simulink model "RadarSimulinkProjectRev011"  (R2024a)
settings: Solver=VariableStepAuto  StartTime=0.0  StopTime=0.0125*2  RelTol=1e-3
values from neighbouring files (symbols this model uses):
  AngleTime = SweepTime/10    (= 10000)    [InitializationOfVariablesRev000.m]    (also in InitializationOfVariablesRev001.m; InitializationOfVariablesRev002.m = 2000; InitializationOfVariablesRev003.m = 20000; InitializationOfVariablesRev004.m = 2097152)
  ASR_LUT = Rsamp    [InitializationOfVariablesRev003.m]    (also in InitializationOfVariablesRev004.m = round((R*2*SystemFs)/c); InitializationOfVariablesRev005.m = round((R*2*SystemFs)/c))
  Btn_Debounce = 20000    [InitializationOfVariablesRev003.m]    (also in InitializationOfVariablesRev004.m; InitializationOfVariablesRev005.m)
  ChirpNc = 128    [InitializationOfVariablesRev004.m]    (also in InitializationOfVariablesRev005.m)
  ChirpSizeLength = length(FCW)    [InitializationOfVariablesRev004.m]    (also in InitializationOfVariablesRev005.m = 16384)
  DeciFactor = 8    [InitializationOfVariablesRev005.m]
  FCW = [FCW_p1, FCW_p2]    [InitializationOfVariablesRev002.m]    (also in InitializationOfVariablesRev003.m; InitializationOfVariablesRev004.m = interp1(1:length(FCW_base), FCW_base,      linspace(1, lengt; InitializationOfVariablesRev005.m = f / SystemFs)
  RXFFTLength = 4096    [InitializationOfVariablesRev003.m]    (also in InitializationOfVariablesRev004.m = 1024; InitializationOfVariablesRev005.m = 2048)
  SweepTime = 100000    [InitializationOfVariablesRev000.m]    (also in InitializationOfVariablesRev001.m; InitializationOfVariablesRev002.m = 20000; InitializationOfVariablesRev003.m = 200000; InitializationOfVariablesRev004.m = 23068672)
undefined symbols (not defined in the file or in its folder): SignalGenerationForAnalysis, Subsystem, xc7a200tfbg676
libraries: hdlBasic x453, hdlUtilities x11, hdlDSPIP x11, vmcUtilities x1
(part 4 of 5)

== system RadarSimulinkProjectRev011/RangeProcessing/DC Removal3 ==
  note: Measured delay between DC removal and RAM delay, offset by 54 (apparently)
  DataIN : Inport
  tlast : Inport  Port=2
  tready : Inport  Port=3
  Accumulator : hdlBasic/Accumulator  operation=Add  n_bits=64  overflow=Wrap  scale=1  rst=on  hasbypass=off  en=on  latency=1  msb_inp=100  msb=100  lsb=-100  use_behavioral_HDL=on  implementation=Fabric  XmcBlockStatus=1  maskContainerNames=group3  block_type=accum  block_config=sysgen:Accum_config  block_width=566  block_height=845
  AddSub : hdlBasic/AddSub  mode=Subtraction  use_carryin=off  use_carryout=off  en=off  latency=1  precision=Full  arith_type=Unsigned  n_bits=16  bin_pt=14  quantization=Truncate  overflow=Wrap  use_behavioral_HDL=off  hw_selection=Fabric  pipelined=off  XmcBlockStatus=1  maskContainerNames=tabcontainer1  block_type=addsub  block_config=sysgen:Addsub_config
  Constant : hdlBasic/Constant  const=ChirpSizeLength-1  gui_display_data_type=Fixed-point  arith_type=Signed (2's comp)  n_bits=16  bin_pt=0  preci_type=Single  exp_width=8  frac_width=24  explicit_period=on  period=P1  XmcBlockStatus=1  maskContainerNames=tabcontainer1  block_type=constant  block_config=sysgen:Constant_config
  Constant1 : hdlBasic/Constant  const=ChirpSizeLength-1  gui_display_data_type=Fixed-point  arith_type=Signed (2's comp)  n_bits=16  bin_pt=0  preci_type=Single  exp_width=8  frac_width=24  explicit_period=off  period=1  XmcBlockStatus=1  maskContainerNames=tabcontainer1  block_type=constant  block_config=sysgen:Constant_config
  Convert10 : hdlBasic/Convert  gui_display_data_type=Fixed-point  arith_type=Signed (2's comp)  n_bits=32  bin_pt=16  float_type=Single  exp_bits=8  fraction_bits=24  quantization="Round  (unbiased: Even Values)"  overflow=Saturate  en=off  latency=1  pipeline=off  XmcBlockStatus=1  maskContainerNames=group2  block_type=convert  block_config=sysgen:Convert_config  block_width=595  block_height=885
  Counter : hdlBasic/Counter  cnt_type=Count limited  cnt_to=ChirpSizeLength-1  operation=Up  start_count=0  cnt_by_val=1  arith_type=Unsigned  n_bits=14  bin_pt=0  load_pin=off  rst=on  en=on  explicit_period=Explicit  period=P1  use_behavioral_HDL=off  implementation=Fabric  XmcBlockStatus=1  maskContainerNames=group1  block_type=counter  block_config=sysgen:Counter_config  block_width=531  block_height=1023
  Counter1 : hdlBasic/Counter  cnt_type=Count limited  cnt_to=ChirpSizeLength-1  operation=Up  start_count=0  cnt_by_val=1  arith_type=Unsigned  n_bits=14  bin_pt=0  load_pin=off  rst=on  en=on  explicit_period=Explicit  period=P1  use_behavioral_HDL=off  implementation=Fabric  XmcBlockStatus=1  maskContainerNames=group1  block_type=counter  block_config=sysgen:Counter_config  block_width=531  block_height=1023
  Delay1 : hdlBasic/Delay  rst=off  en=off  latency=72  reg_retiming=off  XmcBlockStatus=1  maskContainerNames=group1  block_type=delay  block_config=sysgen:Delay_config
  Delay2 : hdlBasic/Delay  rst=off  en=off  latency=55  reg_retiming=off  XmcBlockStatus=1  maskContainerNames=group1  block_type=delay  block_config=sysgen:Delay_config
  Divide : hdlBasic/Divide  flow_control=NonBlocking  axi_optimize_goal=Resources  algorithm_type=Radix2  fractional_width=32  latency=1  rate=1  has_a_tlast=off  has_a_tuser=off  has_b_tlast=off  has_b_tuser=off  en=off  has_result_tready=off  result_tlast_behv=Pass_A_TLAST  has_underflow=off  has_overflow=off  has_invalid_op=off  has_divide_by_zero=off  fpo_op_type=mergeddivide  XmcBlockStatus=1  maskContainerNames=tabcontainer1  block_type=divide  block_config=sysgen:FPOBlockDescriptor_config
  Register : hdlBasic/Register  init=0  rst=off  en=on  XmcBlockStatus=1  maskContainerNames=tabcontainer1  block_type=register  block_config=sysgen:Register_config
  Relational : hdlBasic/Relational  mode=a=b  op_type=Bool  en=off  latency=0  XmcBlockStatus=1  maskContainerNames=tabcontainer1  block_type=relational  block_config=sysgen:Relational_config
  Simple Dual Port RAM : hdlBasic/Simple Dual Port RAM  depth=ChirpSizeLength  initVector=0  distributed_mem=Distributed memory  init_b=0  rst_b=off  en_a=off  en_b=off  latency=1  write_mode_B=Read After Write  explicit_period=[]  period=[]  simulation_type=fast_sim  XmcBlockStatus=1  maskContainerNames=tabcontainer1  block_type=sdpram  block_config=sysgen:Sdpram_config  optimize=Area
      settings: infoedit=[]
  Simple Dual Port RAM1 : hdlBasic/Simple Dual Port RAM  depth=ChirpSizeLength  initVector=0  distributed_mem=Distributed memory  init_b=0  rst_b=off  en_a=off  en_b=off  latency=1  write_mode_B=Read After Write  explicit_period=[]  period=[]  simulation_type=fast_sim  XmcBlockStatus=1  maskContainerNames=tabcontainer1  block_type=sdpram  block_config=sysgen:Sdpram_config  optimize=Area
      settings: infoedit=[]
  DataOUT : Outport
  treadyOUT : Outport  Port=2
  wires:
  Accumulator/1 -> Register/1
  Register/1 -> Divide/1
  AddSub/1 -> Convert10/1
  Constant/1 -> Divide/2
  Counter/1 -> Simple Dual Port RAM1/1, Simple Dual Port RAM/1, Relational/2
  Counter1/1 -> Simple Dual Port RAM1/4, Simple Dual Port RAM/4
  Constant1/1 -> Relational/1
  Simple Dual Port RAM/1 -> Delay1/1
  Simple Dual Port RAM1/1 -> Delay2/1
  Delay2/1 -> treadyOUT/1
  Convert10/1 -> DataOUT/1
  Delay1/1 -> AddSub/1
  Divide/1 -> AddSub/2
  DataIN/1 -> Accumulator/1, Simple Dual Port RAM/2
  tready/1 -> Accumulator/3, Counter1/2, Simple Dual Port RAM1/3, Simple Dual Port RAM1/2, Simple Dual Port RAM/3, Counter/2
  tlast/1 -> Register/2, Accumulator/2, Counter/1
  Relational/1 -> Counter1/1

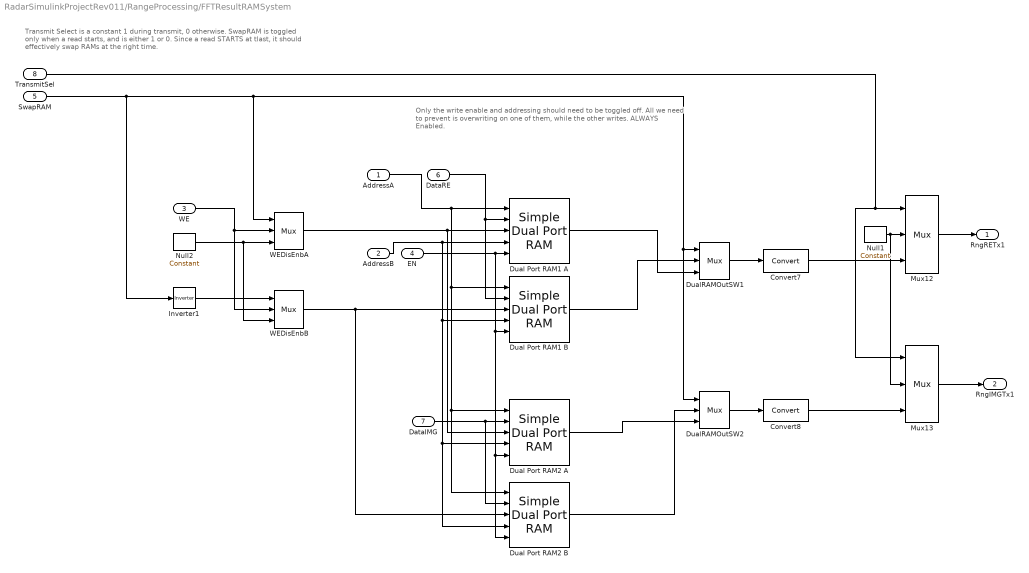
== system RadarSimulinkProjectRev011/RangeProcessing/FFTResultRAMSystem ==
  note: Transmit Select is a constant 1 during transmit, 0 otherwise.
      | SwapRAM is toggled only when a read starts, and is either 1 or 0.
      | Since a read STARTS at tlast, it should effectively swap RAMs at the right time.
  note: Only the write enable and addressing should need to be toggled off.
      | All we need to prevent is overwriting on one of them, while the other writes.
      | ALWAYS Enabled.
  AddressA : Inport
  AddressB : Inport  Port=2
  WE : Inport  Port=3
  EN : Inport  Port=4
  SwapRAM : Inport  Port=5
  DataRE : Inport  Port=6
  DataIMG : Inport  Port=7
  TransmitSel : Inport  Port=8
  Convert7 : hdlBasic/Convert  gui_display_data_type=Fixed-point  arith_type="Signed  (2's comp)"  n_bits=17  bin_pt=16  float_type=Single  exp_bits=8  fraction_bits=24  quantization=Truncate  overflow=Saturate  en=off  latency=0  pipeline=off  XmcBlockStatus=1  maskContainerNames=group2  block_type=convert  block_config=sysgen:Convert_config  block_width=595  block_height=885
  Convert8 : hdlBasic/Convert  gui_display_data_type=Fixed-point  arith_type="Signed  (2's comp)"  n_bits=17  bin_pt=16  float_type=Single  exp_bits=8  fraction_bits=24  quantization=Truncate  overflow=Saturate  en=off  latency=0  pipeline=off  XmcBlockStatus=1  maskContainerNames=group2  block_type=convert  block_config=sysgen:Convert_config  block_width=595  block_height=885
  Dual Port RAM1 A : hdlBasic/Simple Dual Port RAM  depth=ChirpNc*RXFFTLength  initVector=0  distributed_mem=Distributed memory  init_b=0  rst_b=off  en_a=on  en_b=off  latency=1  write_mode_B=Read After Write  explicit_period=[]  period=[]  simulation_type=fast_sim  XmcBlockStatus=1  maskContainerNames=tabcontainer1  block_type=sdpram  block_config=sysgen:Sdpram_config  optimize=Area
      settings: infoedit=[]
  Dual Port RAM1 B : hdlBasic/Simple Dual Port RAM  depth=ChirpNc*RXFFTLength  initVector=0  distributed_mem=Distributed memory  init_b=0  rst_b=off  en_a=on  en_b=off  latency=1  write_mode_B=Read After Write  explicit_period=[]  period=[]  simulation_type=fast_sim  XmcBlockStatus=1  maskContainerNames=tabcontainer1  block_type=sdpram  block_config=sysgen:Sdpram_config  optimize=Area
      settings: infoedit=[]
  Dual Port RAM2 A : hdlBasic/Simple Dual Port RAM  depth=ChirpNc*RXFFTLength  initVector=0  distributed_mem=Distributed memory  init_b=0  rst_b=off  en_a=on  en_b=off  latency=1  write_mode_B=Read After Write  explicit_period=[]  period=[]  simulation_type=fast_sim  XmcBlockStatus=1  maskContainerNames=tabcontainer1  block_type=sdpram  block_config=sysgen:Sdpram_config  optimize=Area
      settings: infoedit=[]
  Dual Port RAM2 B : hdlBasic/Simple Dual Port RAM  depth=ChirpNc*RXFFTLength  initVector=0  distributed_mem=Distributed memory  init_b=0  rst_b=off  en_a=on  en_b=off  latency=1  write_mode_B=Read After Write  explicit_period=[]  period=[]  simulation_type=fast_sim  XmcBlockStatus=1  maskContainerNames=tabcontainer1  block_type=sdpram  block_config=sysgen:Sdpram_config  optimize=Area
      settings: infoedit=[]
  DualRAMOutSW1 : hdlBasic/Mux  inputs=2  en=off  latency=0  precision=Full  arith_type=Unsigned  n_bits=16  bin_pt=14  quantization=Truncate  overflow=Wrap  XmcBlockStatus=1  maskContainerNames=tabcontainer1  block_type=mux  block_config=sysgen:Mux_config
  DualRAMOutSW2 : hdlBasic/Mux  inputs=2  en=off  latency=0  precision=Full  arith_type=Unsigned  n_bits=16  bin_pt=14  quantization=Truncate  overflow=Wrap  XmcBlockStatus=1  maskContainerNames=tabcontainer1  block_type=mux  block_config=sysgen:Mux_config
  Inverter1 : hdlBasic/Inverter  en=off  latency=0  XmcBlockStatus=1  maskContainerNames=group2  block_type=inv  block_config=sysgen:Inverter_config
  Mux12 : hdlBasic/Mux  inputs=2  en=off  latency=0  precision=Full  arith_type=Unsigned  n_bits=16  bin_pt=14  quantization=Truncate  overflow=Wrap  XmcBlockStatus=1  maskContainerNames=tabcontainer1  block_type=mux  block_config=sysgen:Mux_config
  Mux13 : hdlBasic/Mux  inputs=2  en=off  latency=0  precision=Full  arith_type=Unsigned  n_bits=16  bin_pt=14  quantization=Truncate  overflow=Wrap  XmcBlockStatus=1  maskContainerNames=tabcontainer1  block_type=mux  block_config=sysgen:Mux_config
  Null1 : hdlBasic/Constant  const=0  gui_display_data_type=Fixed-point  arith_type=Signed (2's comp)  n_bits=16  bin_pt=15  preci_type=Single  exp_width=8  frac_width=24  explicit_period=on  period=P2  XmcBlockStatus=1  maskContainerNames=tabcontainer1  block_type=constant  block_config=sysgen:Constant_config
  Null2 : hdlBasic/Constant  const=0  gui_display_data_type=Boolean  arith_type=Boolean  n_bits=16  bin_pt=15  preci_type=Single  exp_width=8  frac_width=24  explicit_period=on  period=P2  XmcBlockStatus=1  maskContainerNames=tabcontainer1  block_type=constant  block_config=sysgen:Constant_config
  WEDisEnbA : hdlBasic/Mux  inputs=2  en=off  latency=0  precision=Full  arith_type=Unsigned  n_bits=16  bin_pt=14  quantization=Truncate  overflow=Wrap  XmcBlockStatus=1  maskContainerNames=tabcontainer1  block_type=mux  block_config=sysgen:Mux_config
  WEDisEnbB : hdlBasic/Mux  inputs=2  en=off  latency=0  precision=Full  arith_type=Unsigned  n_bits=16  bin_pt=14  quantization=Truncate  overflow=Wrap  XmcBlockStatus=1  maskContainerNames=tabcontainer1  block_type=mux  block_config=sysgen:Mux_config
  RngRETx1 : Outport
  RngIMGTx1 : Outport  Port=2
  wires:
  Mux13/1 -> RngIMGTx1/1
  Mux12/1 -> RngRETx1/1
  Convert8/1 -> Mux13/3
  Convert7/1 -> Mux12/3
  TransmitSel/1 -> Mux12/1, Mux13/1
  Dual Port RAM2 A/1 -> DualRAMOutSW2/3
  Dual Port RAM1 A/1 -> DualRAMOutSW1/3
  Null1/1 -> Mux13/2, Mux12/2
  Dual Port RAM1 B/1 -> DualRAMOutSW1/2
  DualRAMOutSW1/1 -> Convert7/1
  DataRE/1 -> Dual Port RAM1 B/2, Dual Port RAM1 A/2
  DataIMG/1 -> Dual Port RAM2 B/2, Dual Port RAM2 A/2
  EN/1 -> Dual Port RAM1 A/5, Dual Port RAM1 B/5, Dual Port RAM2 B/5, Dual Port RAM2 A/5
  Null2/1 -> WEDisEnbB/3, WEDisEnbA/3
  Dual Port RAM2 B/1 -> DualRAMOutSW2/2
  DualRAMOutSW2/1 -> Convert8/1
  WE/1 -> WEDisEnbB/2, WEDisEnbA/2
  AddressA/1 -> Dual Port RAM1 A/1, Dual Port RAM1 B/1, Dual Port RAM2 A/1, Dual Port RAM2 B/1
  AddressB/1 -> Dual Port RAM2 A/4, Dual Port RAM2 B/4, Dual Port RAM1 B/4, Dual Port RAM1 A/4
  Inverter1/1 -> WEDisEnbB/1
  SwapRAM/1 -> Inverter1/1, WEDisEnbA/1, DualRAMOutSW2/1, DualRAMOutSW1/1
  WEDisEnbA/1 -> Dual Port RAM2 A/3, Dual Port RAM1 A/3
  WEDisEnbB/1 -> Dual Port RAM2 B/3, Dual Port RAM1 B/3

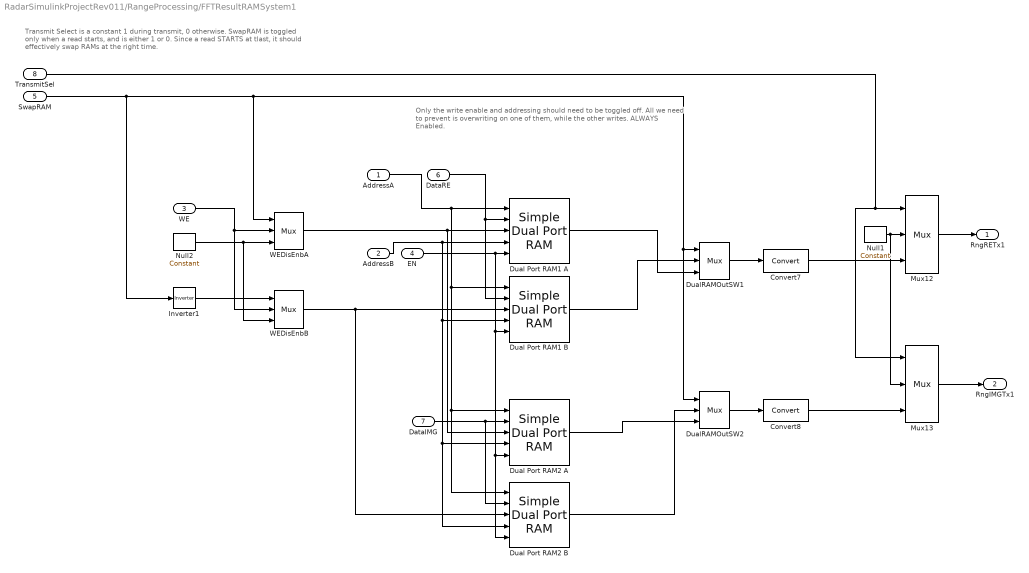
== system RadarSimulinkProjectRev011/RangeProcessing/FFTResultRAMSystem1 ==
  note: Transmit Select is a constant 1 during transmit, 0 otherwise.
      | SwapRAM is toggled only when a read starts, and is either 1 or 0.
      | Since a read STARTS at tlast, it should effectively swap RAMs at the right time.
  note: Only the write enable and addressing should need to be toggled off.
      | All we need to prevent is overwriting on one of them, while the other writes.
      | ALWAYS Enabled.
  AddressA : Inport
  AddressB : Inport  Port=2
  WE : Inport  Port=3
  EN : Inport  Port=4
  SwapRAM : Inport  Port=5
  DataRE : Inport  Port=6
  DataIMG : Inport  Port=7
  TransmitSel : Inport  Port=8
  Convert7 : hdlBasic/Convert  gui_display_data_type=Fixed-point  arith_type="Signed  (2's comp)"  n_bits=17  bin_pt=16  float_type=Single  exp_bits=8  fraction_bits=24  quantization=Truncate  overflow=Saturate  en=off  latency=0  pipeline=off  XmcBlockStatus=1  maskContainerNames=group2  block_type=convert  block_config=sysgen:Convert_config  block_width=595  block_height=885
  Convert8 : hdlBasic/Convert  gui_display_data_type=Fixed-point  arith_type="Signed  (2's comp)"  n_bits=17  bin_pt=16  float_type=Single  exp_bits=8  fraction_bits=24  quantization=Truncate  overflow=Saturate  en=off  latency=0  pipeline=off  XmcBlockStatus=1  maskContainerNames=group2  block_type=convert  block_config=sysgen:Convert_config  block_width=595  block_height=885
  Dual Port RAM1 A : hdlBasic/Simple Dual Port RAM  depth=ChirpNc*RXFFTLength  initVector=0  distributed_mem=Distributed memory  init_b=0  rst_b=off  en_a=on  en_b=off  latency=1  write_mode_B=Read After Write  explicit_period=[]  period=[]  simulation_type=fast_sim  XmcBlockStatus=1  maskContainerNames=tabcontainer1  block_type=sdpram  block_config=sysgen:Sdpram_config  optimize=Area
      settings: infoedit=[]
  Dual Port RAM1 B : hdlBasic/Simple Dual Port RAM  depth=ChirpNc*RXFFTLength  initVector=0  distributed_mem=Distributed memory  init_b=0  rst_b=off  en_a=on  en_b=off  latency=1  write_mode_B=Read After Write  explicit_period=[]  period=[]  simulation_type=fast_sim  XmcBlockStatus=1  maskContainerNames=tabcontainer1  block_type=sdpram  block_config=sysgen:Sdpram_config  optimize=Area
      settings: infoedit=[]
  Dual Port RAM2 A : hdlBasic/Simple Dual Port RAM  depth=ChirpNc*RXFFTLength  initVector=0  distributed_mem=Distributed memory  init_b=0  rst_b=off  en_a=on  en_b=off  latency=1  write_mode_B=Read After Write  explicit_period=[]  period=[]  simulation_type=fast_sim  XmcBlockStatus=1  maskContainerNames=tabcontainer1  block_type=sdpram  block_config=sysgen:Sdpram_config  optimize=Area
      settings: infoedit=[]
  Dual Port RAM2 B : hdlBasic/Simple Dual Port RAM  depth=ChirpNc*RXFFTLength  initVector=0  distributed_mem=Distributed memory  init_b=0  rst_b=off  en_a=on  en_b=off  latency=1  write_mode_B=Read After Write  explicit_period=[]  period=[]  simulation_type=fast_sim  XmcBlockStatus=1  maskContainerNames=tabcontainer1  block_type=sdpram  block_config=sysgen:Sdpram_config  optimize=Area
      settings: infoedit=[]
  DualRAMOutSW1 : hdlBasic/Mux  inputs=2  en=off  latency=0  precision=Full  arith_type=Unsigned  n_bits=16  bin_pt=14  quantization=Truncate  overflow=Wrap  XmcBlockStatus=1  maskContainerNames=tabcontainer1  block_type=mux  block_config=sysgen:Mux_config
  DualRAMOutSW2 : hdlBasic/Mux  inputs=2  en=off  latency=0  precision=Full  arith_type=Unsigned  n_bits=16  bin_pt=14  quantization=Truncate  overflow=Wrap  XmcBlockStatus=1  maskContainerNames=tabcontainer1  block_type=mux  block_config=sysgen:Mux_config
  Inverter1 : hdlBasic/Inverter  en=off  latency=0  XmcBlockStatus=1  maskContainerNames=group2  block_type=inv  block_config=sysgen:Inverter_config
  Mux12 : hdlBasic/Mux  inputs=2  en=off  latency=0  precision=Full  arith_type=Unsigned  n_bits=16  bin_pt=14  quantization=Truncate  overflow=Wrap  XmcBlockStatus=1  maskContainerNames=tabcontainer1  block_type=mux  block_config=sysgen:Mux_config
  Mux13 : hdlBasic/Mux  inputs=2  en=off  latency=0  precision=Full  arith_type=Unsigned  n_bits=16  bin_pt=14  quantization=Truncate  overflow=Wrap  XmcBlockStatus=1  maskContainerNames=tabcontainer1  block_type=mux  block_config=sysgen:Mux_config
  Null1 : hdlBasic/Constant  const=0  gui_display_data_type=Fixed-point  arith_type=Signed (2's comp)  n_bits=16  bin_pt=15  preci_type=Single  exp_width=8  frac_width=24  explicit_period=on  period=P2  XmcBlockStatus=1  maskContainerNames=tabcontainer1  block_type=constant  block_config=sysgen:Constant_config
  Null2 : hdlBasic/Constant  const=0  gui_display_data_type=Boolean  arith_type=Boolean  n_bits=16  bin_pt=15  preci_type=Single  exp_width=8  frac_width=24  explicit_period=on  period=P2  XmcBlockStatus=1  maskContainerNames=tabcontainer1  block_type=constant  block_config=sysgen:Constant_config
  WEDisEnbA : hdlBasic/Mux  inputs=2  en=off  latency=0  precision=Full  arith_type=Unsigned  n_bits=16  bin_pt=14  quantization=Truncate  overflow=Wrap  XmcBlockStatus=1  maskContainerNames=tabcontainer1  block_type=mux  block_config=sysgen:Mux_config
  WEDisEnbB : hdlBasic/Mux  inputs=2  en=off  latency=0  precision=Full  arith_type=Unsigned  n_bits=16  bin_pt=14  quantization=Truncate  overflow=Wrap  XmcBlockStatus=1  maskContainerNames=tabcontainer1  block_type=mux  block_config=sysgen:Mux_config
  RngRETx1 : Outport
  RngIMGTx1 : Outport  Port=2
  wires:
  Mux13/1 -> RngIMGTx1/1
  Mux12/1 -> RngRETx1/1
  Convert8/1 -> Mux13/3
  Convert7/1 -> Mux12/3
  TransmitSel/1 -> Mux12/1, Mux13/1
  Dual Port RAM2 A/1 -> DualRAMOutSW2/3
  Dual Port RAM1 A/1 -> DualRAMOutSW1/3
  Null1/1 -> Mux13/2, Mux12/2
  Dual Port RAM1 B/1 -> DualRAMOutSW1/2
  DualRAMOutSW1/1 -> Convert7/1
  DataRE/1 -> Dual Port RAM1 B/2, Dual Port RAM1 A/2
  DataIMG/1 -> Dual Port RAM2 B/2, Dual Port RAM2 A/2
  EN/1 -> Dual Port RAM1 A/5, Dual Port RAM1 B/5, Dual Port RAM2 B/5, Dual Port RAM2 A/5
  Null2/1 -> WEDisEnbB/3, WEDisEnbA/3
  Dual Port RAM2 B/1 -> DualRAMOutSW2/2
  DualRAMOutSW2/1 -> Convert8/1
  WE/1 -> WEDisEnbB/2, WEDisEnbA/2
  AddressA/1 -> Dual Port RAM1 A/1, Dual Port RAM1 B/1, Dual Port RAM2 A/1, Dual Port RAM2 B/1
  AddressB/1 -> Dual Port RAM2 A/4, Dual Port RAM2 B/4, Dual Port RAM1 B/4, Dual Port RAM1 A/4
  Inverter1/1 -> WEDisEnbB/1
  SwapRAM/1 -> Inverter1/1, WEDisEnbA/1, DualRAMOutSW2/1, DualRAMOutSW1/1
  WEDisEnbA/1 -> Dual Port RAM2 A/3, Dual Port RAM1 A/3
  WEDisEnbB/1 -> Dual Port RAM2 B/3, Dual Port RAM1 B/3

== system RadarSimulinkProjectRev011/RangeProcessing/FFTTracking ==
  note: Should restart counter at beggining or end,
      | In Radix mode, Tlast is not the beggining because there is a gap
  note: In Radix burst, this is active for only real frame of data
      | In Pipeline, it's always active
  note: Bring back to 0 at start
  note: Only count for valid FFT points of data
      | Note: Add reset later
  data_Active : Inport
  StatusReady : Inport  Port=2
  DecimatedTrig : Inport  Port=3
  AddrforIQvals : hdlBasic/Counter  cnt_type=Count limited  cnt_to=ChirpNc*RXFFTLength-1  operation=Up  start_count=0  cnt_by_val=1  arith_type=Unsigned  n_bits=18  bin_pt=0  load_pin=off  rst=off  en=on  explicit_period=Explicit  period=P1  use_behavioral_HDL=off  implementation=Fabric  XmcBlockStatus=1  maskContainerNames=group1  block_type=counter  block_config=sysgen:Counter_config  block_width=531  block_height=1023
  ChirpSamples : hdlBasic/Constant  const=ChirpSizeLength/2-1  gui_display_data_type=Fixed-point  arith_type=Unsigned  n_bits=13  bin_pt=0  preci_type=Single  exp_width=8  frac_width=24  explicit_period=on  period=P2  XmcBlockStatus=1  maskContainerNames=tabcontainer1  block_type=constant  block_config=sysgen:Constant_config
  Counter2 : hdlBasic/Counter  cnt_type=Count limited  cnt_to=ChirpSizeLength-1  operation=Up  start_count=0  cnt_by_val=1  arith_type=Unsigned  n_bits=14  bin_pt=0  load_pin=off  rst=off  en=on  explicit_period=Explicit  period=P1  use_behavioral_HDL=off  implementation=Fabric  XmcBlockStatus=1  maskContainerNames=group1  block_type=counter  block_config=sysgen:Counter_config  block_width=531  block_height=1023
  Delay : hdlBasic/Delay  rst=off  en=off  latency=4  reg_retiming=off  XmcBlockStatus=1  maskContainerNames=group1  block_type=delay  block_config=sysgen:Delay_config
  FFTSamplingRelation : hdlBasic/Relational  mode=a<=b  op_type=Bool  en=off  latency=0  XmcBlockStatus=1  maskContainerNames=tabcontainer1  block_type=relational  block_config=sysgen:Relational_config
  Gateway Out1 : hdlBasic/Gateway Out  inherit_from_input=off  bool_to_boolean=off  hdl_port=on  rows=1  columns=1  UseAsDAC=off  DACChannel='1'  interface=None  automatic_assignment=on  address_offset=hex2dec('00')  intf_name=''  intf_description=''  timing_constraint=None  locs_specified=off  LOCs={}  io_standard={}  XmcBlockStatus=1  maskContainerNames=group4  block_type=gatewayout  block_config=sysgen:gateway_out_config  block_width_w=590  block_height_w=620  block_width=620  block_height=750
  Gateway Out15 : hdlBasic/Gateway Out  inherit_from_input=off  bool_to_boolean=off  hdl_port=on  rows=1  columns=1  UseAsDAC=off  DACChannel='1'  interface=None  automatic_assignment=on  address_offset=hex2dec('00')  intf_name=''  intf_description=''  timing_constraint=None  locs_specified=off  LOCs={}  io_standard={}  XmcBlockStatus=1  maskContainerNames=group4  block_type=gatewayout  block_config=sysgen:gateway_out_config  block_width_w=590  block_height_w=620  block_width=620  block_height=750
  Gateway Out4 : hdlBasic/Gateway Out  inherit_from_input=off  bool_to_boolean=off  hdl_port=on  rows=1  columns=1  UseAsDAC=off  DACChannel='1'  interface=None  automatic_assignment=on  address_offset=hex2dec('00')  intf_name=''  intf_description=''  timing_constraint=None  locs_specified=off  LOCs={}  io_standard={}  XmcBlockStatus=1  maskContainerNames=group4  block_type=gatewayout  block_config=sysgen:gateway_out_config  block_width_w=590  block_height_w=620  block_width=620  block_height=750
  IndexTracker : hdlBasic/Counter  cnt_type=Count limited  cnt_to=RXFFTLength*DeciFactor-1  operation=Up  start_count=0  cnt_by_val=1  arith_type=Unsigned  n_bits=14  bin_pt=0  load_pin=off  rst=on  en=on  explicit_period=Explicit  period=P1  use_behavioral_HDL=off  implementation=Fabric  XmcBlockStatus=1  maskContainerNames=group1  block_type=counter  block_config=sysgen:Counter_config  block_width=531  block_height=1023
  Inverter : hdlBasic/Inverter  en=off  latency=0  XmcBlockStatus=1  maskContainerNames=group2  block_type=inv  block_config=sysgen:Inverter_config
  Logical1 : hdlBasic/Logical  logical_function=AND  inputs=2  en=off  latency=0  precision=Full  arith_type=Unsigned  n_bits=16  bin_pt=0  align_bp=on  overflow=[]  quantization=[]  XmcBlockStatus=1  maskContainerNames=tabcontainer1  block_type=logical  block_config=sysgen:Logical_config
  Logical2 : hdlBasic/Logical  logical_function=AND  inputs=2  en=off  latency=0  precision=Full  arith_type=Unsigned  n_bits=16  bin_pt=0  align_bp=on  overflow=[]  quantization=[]  XmcBlockStatus=1  maskContainerNames=tabcontainer1  block_type=logical  block_config=sysgen:Logical_config
  Scope3 : Scope  NumInputPorts=3
  FFTIndex : Outport
  PeakSerachEnable : Outport  Port=2
  IQDataADDR : Outport  Port=3
  wires:
  IndexTracker/1 -> FFTIndex/1
  Inverter/1 -> IndexTracker/1
  DecimatedTrig/1 -> Gateway Out15/1, Logical2/1
  Logical1/1 -> Delay/1
  StatusReady/1 -> Logical1/1, Inverter/1
  data_Active/1 -> Logical2/2, Logical1/2
  AddrforIQvals/1 -> Gateway Out1/1, IQDataADDR/1
  Logical2/1 -> AddrforIQvals/1
  Gateway Out15/1 -> Scope3/3
  Gateway Out1/1 -> Scope3/2
  Gateway Out4/1 -> Scope3/1
  ChirpSamples/1 -> FFTSamplingRelation/2
  Counter2/1 -> FFTSamplingRelation/1
  FFTSamplingRelation/1 -> Gateway Out4/1, PeakSerachEnable/1  "TLast"
  Delay/1 -> Counter2/1, IndexTracker/2

== system RadarSimulinkProjectRev011/RangeProcessing/ManualDownsample1 ==
  data_valid : Inport
  IMGin : Inport  Port=2
  REin : Inport  Port=3
  Constant1 : hdlBasic/Constant  const=RXFFTLength*8-1  gui_display_data_type=Fixed-point  arith_type=Signed (2's comp)  n_bits=16  bin_pt=0  preci_type=Single  exp_width=8  frac_width=24  explicit_period=off  period=1  XmcBlockStatus=1  maskContainerNames=tabcontainer1  block_type=constant  block_config=sysgen:Constant_config
  Delay : hdlBasic/Delay  rst=off  en=off  latency=1  reg_retiming=off  XmcBlockStatus=1  maskContainerNames=group1  block_type=delay  block_config=sysgen:Delay_config
  FFTSampler : hdlBasic/Counter  cnt_type=Count limited  cnt_to=DeciFactor-1  operation=Up  start_count=0  cnt_by_val=1  arith_type=Unsigned  n_bits=4  bin_pt=0  load_pin=off  rst=off  en=on  explicit_period=Explicit  period=P1  use_behavioral_HDL=off  implementation=Fabric  XmcBlockStatus=1  maskContainerNames=group1  block_type=counter  block_config=sysgen:Counter_config  block_width=531  block_height=1023
  Register : hdlBasic/Register  init=0  rst=on  en=on  XmcBlockStatus=1  maskContainerNames=tabcontainer1  block_type=register  block_config=sysgen:Register_config
  Register1 : hdlBasic/Register  init=0  rst=on  en=on  XmcBlockStatus=1  maskContainerNames=tabcontainer1  block_type=register  block_config=sysgen:Register_config
  Relational1 : hdlBasic/Relational  mode=a=b  op_type=Bool  en=off  latency=0  XmcBlockStatus=1  maskContainerNames=tabcontainer1  block_type=relational  block_config=sysgen:Relational_config
  SamNum : hdlBasic/Constant  const=0  gui_display_data_type=Fixed-point  arith_type=Signed (2's comp)  n_bits=5  bin_pt=0  preci_type=Single  exp_width=8  frac_width=24  explicit_period=off  period=1  XmcBlockStatus=1  maskContainerNames=tabcontainer1  block_type=constant  block_config=sysgen:Constant_config
  TlastDecimated : hdlBasic/Counter  cnt_type=Count limited  cnt_to=2047  operation=Up  start_count=0  cnt_by_val=1  arith_type=Unsigned  n_bits=12  bin_pt=0  load_pin=off  rst=off  en=on  explicit_period=Inferred from inputs  period=P1  use_behavioral_HDL=off  implementation=Fabric  XmcBlockStatus=1  maskContainerNames=group1  block_type=counter  block_config=sysgen:Counter_config  block_width=531  block_height=1023
  datavalidFFT : hdlBasic/Relational  mode=a=b  op_type=Bool  en=off  latency=0  XmcBlockStatus=1  maskContainerNames=tabcontainer1  block_type=relational  block_config=sysgen:Relational_config
  IMG : Outport
  RE : Outport  Port=2
  OnDataTrig : Outport  Port=3
  PassIMG : Outport  Port=4
  PassRE : Outport  Port=5
  wires:
  data_valid/1 -> FFTSampler/1, TlastDecimated/1
  Constant1/1 -> Relational1/1
  FFTSampler/1 -> datavalidFFT/2
  datavalidFFT/1 -> Register1/3, Register/3, Delay/1  "3"
  TlastDecimated/1 -> Relational1/2
  SamNum/1 -> datavalidFFT/1
  Register/1 -> IMG/1
  Register1/1 -> RE/1
  Delay/1 -> OnDataTrig/1
  IMGin/1 -> PassIMG/1, Register/1
  REin/1 -> PassRE/1, Register1/1
  Relational1/1 -> Register/2, Register1/2

== system RadarSimulinkProjectRev011/RangeProcessing/ManualDownsample2 ==
  data_valid : Inport
  IMGin : Inport  Port=2
  REin : Inport  Port=3
  Constant1 : hdlBasic/Constant  const=RXFFTLength*8-1  gui_display_data_type=Fixed-point  arith_type=Signed (2's comp)  n_bits=16  bin_pt=0  preci_type=Single  exp_width=8  frac_width=24  explicit_period=off  period=1  XmcBlockStatus=1  maskContainerNames=tabcontainer1  block_type=constant  block_config=sysgen:Constant_config
  Delay : hdlBasic/Delay  rst=off  en=off  latency=1  reg_retiming=off  XmcBlockStatus=1  maskContainerNames=group1  block_type=delay  block_config=sysgen:Delay_config
  FFTSampler : hdlBasic/Counter  cnt_type=Count limited  cnt_to=DeciFactor-1  operation=Up  start_count=0  cnt_by_val=1  arith_type=Unsigned  n_bits=4  bin_pt=0  load_pin=off  rst=off  en=on  explicit_period=Explicit  period=P1  use_behavioral_HDL=off  implementation=Fabric  XmcBlockStatus=1  maskContainerNames=group1  block_type=counter  block_config=sysgen:Counter_config  block_width=531  block_height=1023
  Register : hdlBasic/Register  init=0  rst=on  en=on  XmcBlockStatus=1  maskContainerNames=tabcontainer1  block_type=register  block_config=sysgen:Register_config
  Register1 : hdlBasic/Register  init=0  rst=on  en=on  XmcBlockStatus=1  maskContainerNames=tabcontainer1  block_type=register  block_config=sysgen:Register_config
  Relational1 : hdlBasic/Relational  mode=a=b  op_type=Bool  en=off  latency=0  XmcBlockStatus=1  maskContainerNames=tabcontainer1  block_type=relational  block_config=sysgen:Relational_config
  SamNum : hdlBasic/Constant  const=0  gui_display_data_type=Fixed-point  arith_type=Signed (2's comp)  n_bits=5  bin_pt=0  preci_type=Single  exp_width=8  frac_width=24  explicit_period=off  period=1  XmcBlockStatus=1  maskContainerNames=tabcontainer1  block_type=constant  block_config=sysgen:Constant_config
  TlastDecimated : hdlBasic/Counter  cnt_type=Count limited  cnt_to=2047  operation=Up  start_count=0  cnt_by_val=1  arith_type=Unsigned  n_bits=12  bin_pt=0  load_pin=off  rst=off  en=on  explicit_period=Inferred from inputs  period=P1  use_behavioral_HDL=off  implementation=Fabric  XmcBlockStatus=1  maskContainerNames=group1  block_type=counter  block_config=sysgen:Counter_config  block_width=531  block_height=1023
  datavalidFFT : hdlBasic/Relational  mode=a=b  op_type=Bool  en=off  latency=0  XmcBlockStatus=1  maskContainerNames=tabcontainer1  block_type=relational  block_config=sysgen:Relational_config
  IMG : Outport
  RE : Outport  Port=2
  OnDataTrig : Outport  Port=3
  PassIMG : Outport  Port=4
  PassRE : Outport  Port=5
  wires:
  data_valid/1 -> FFTSampler/1, TlastDecimated/1
  Constant1/1 -> Relational1/1
  FFTSampler/1 -> datavalidFFT/2
  datavalidFFT/1 -> Register1/3, Register/3, Delay/1  "3"
  TlastDecimated/1 -> Relational1/2
  SamNum/1 -> datavalidFFT/1
  Register/1 -> IMG/1
  Register1/1 -> RE/1
  Delay/1 -> OnDataTrig/1
  IMGin/1 -> PassIMG/1, Register/1
  REin/1 -> PassRE/1, Register1/1
  Relational1/1 -> Register/2, Register1/2

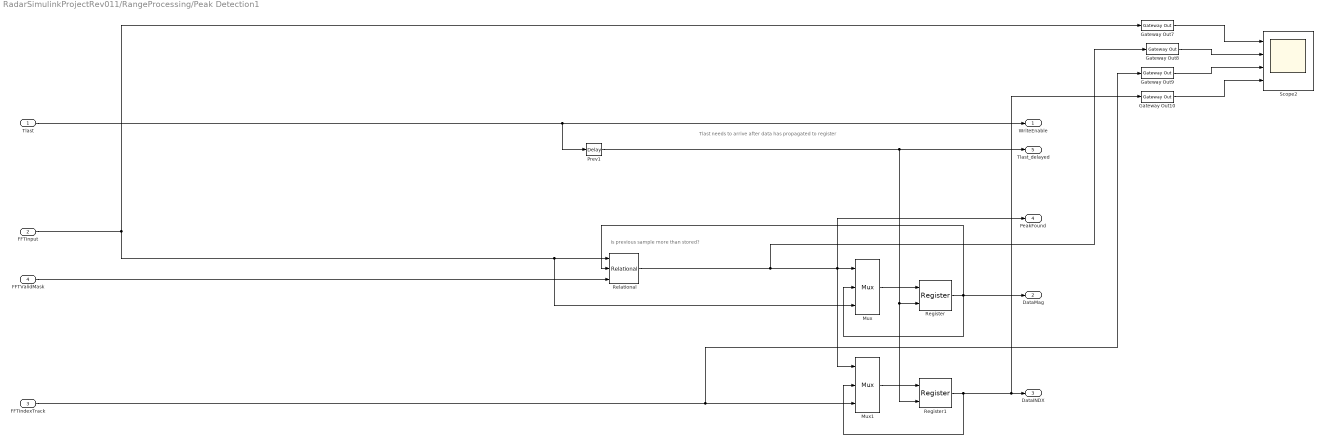
== system RadarSimulinkProjectRev011/RangeProcessing/Peak Detection1 ==
  note: Tlast needs to arrive after data has propagated to register
  note: Is previous sample more than stored?
  Tlast : Inport
  FFTInput : Inport  Port=2
  FFTIndexTrack : Inport  Port=3
  FFTValidMask : Inport  Port=4
  Gateway Out{7..10} (4 alike) : hdlBasic/Gateway Out  inherit_from_input=off  bool_to_boolean=off  hdl_port=on  rows=1  columns=1  UseAsDAC=off  DACChannel='1'  interface=None  automatic_assignment=on  address_offset=hex2dec('00')  intf_name=''  intf_description=''  timing_constraint=None  locs_specified=off  LOCs={}  io_standard={}  XmcBlockStatus=1  maskContainerNames=group4  block_type=gatewayout  block_config=sysgen:gateway_out_config  block_width_w=590  block_height_w=620  block_width=620  block_height=750
  Mux : hdlBasic/Mux  inputs=2  en=off  latency=0  precision=Full  arith_type=Unsigned  n_bits=16  bin_pt=14  quantization=Truncate  overflow=Wrap  XmcBlockStatus=1  maskContainerNames=tabcontainer1  block_type=mux  block_config=sysgen:Mux_config
  Mux1 : hdlBasic/Mux  inputs=2  en=off  latency=0  precision=Full  arith_type=Unsigned  n_bits=16  bin_pt=14  quantization=Truncate  overflow=Wrap  XmcBlockStatus=1  maskContainerNames=tabcontainer1  block_type=mux  block_config=sysgen:Mux_config
  Prev1 : hdlBasic/Delay  rst=off  en=off  latency=4  reg_retiming=off  XmcBlockStatus=1  maskContainerNames=group1  block_type=delay  block_config=sysgen:Delay_config
  Register : hdlBasic/Register  init=0  rst=on  en=off  XmcBlockStatus=1  maskContainerNames=tabcontainer1  block_type=register  block_config=sysgen:Register_config
  Register1 : hdlBasic/Register  init=0  rst=on  en=off  XmcBlockStatus=1  maskContainerNames=tabcontainer1  block_type=register  block_config=sysgen:Register_config
  Relational : hdlBasic/Relational  mode=a>b  op_type=Bool  en=on  latency=1  XmcBlockStatus=1  maskContainerNames=tabcontainer1  block_type=relational  block_config=sysgen:Relational_config
  Scope2 : Scope  NumInputPorts=4
  WriteEnable : Outport
  DataMag : Outport  Port=2
  DataINDX : Outport  Port=3
  PeakFound : Outport  Port=4
  Tlast_delayed : Outport  Port=5
  wires:
  FFTValidMask/1 -> Relational/3
  Tlast/1 -> Prev1/1, WriteEnable/1
  FFTInput/1 -> Gateway Out7/1, Mux/3, Relational/1
  Register/1 -> Relational/2, DataMag/1, Mux/2
  Mux/1 -> Register/1
  Register1/1 -> Gateway Out10/1, DataINDX/1, Mux1/2
  FFTIndexTrack/1 -> Gateway Out9/1, Mux1/3
  Mux1/1 -> Register1/1
  Prev1/1 -> Register1/2, Register/2, Tlast_delayed/1
  Gateway Out7/1 -> Scope2/1
  Gateway Out8/1 -> Scope2/2
  Gateway Out9/1 -> Scope2/3
  Gateway Out10/1 -> Scope2/4
  Relational/1 -> Gateway Out8/1, Mux1/1, Mux/1, PeakFound/1

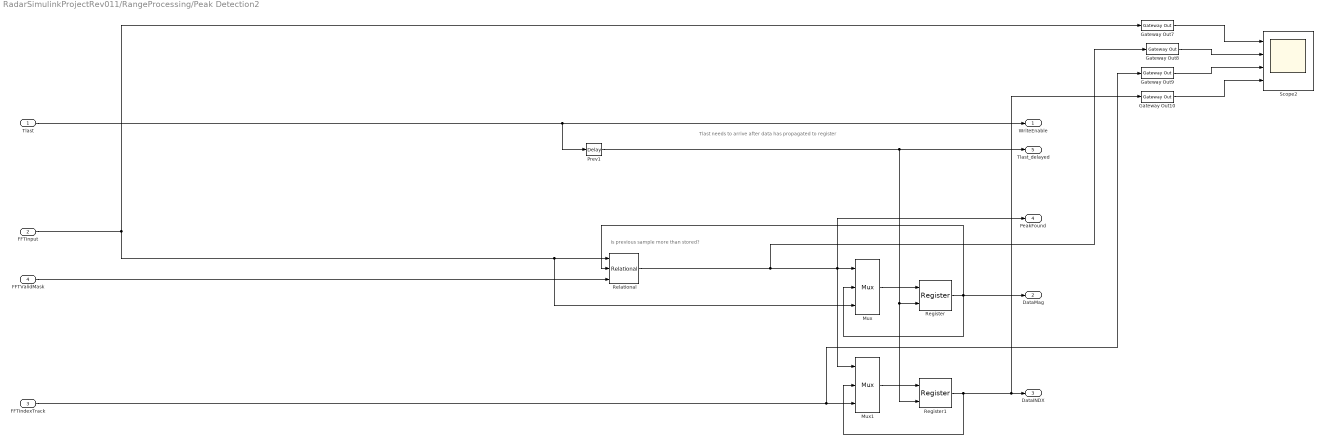
== system RadarSimulinkProjectRev011/RangeProcessing/Peak Detection2 ==
  note: Tlast needs to arrive after data has propagated to register
  note: Is previous sample more than stored?
  Tlast : Inport
  FFTInput : Inport  Port=2
  FFTIndexTrack : Inport  Port=3
  FFTValidMask : Inport  Port=4
  Gateway Out{7..10} (4 alike) : hdlBasic/Gateway Out  inherit_from_input=off  bool_to_boolean=off  hdl_port=on  rows=1  columns=1  UseAsDAC=off  DACChannel='1'  interface=None  automatic_assignment=on  address_offset=hex2dec('00')  intf_name=''  intf_description=''  timing_constraint=None  locs_specified=off  LOCs={}  io_standard={}  XmcBlockStatus=1  maskContainerNames=group4  block_type=gatewayout  block_config=sysgen:gateway_out_config  block_width_w=590  block_height_w=620  block_width=620  block_height=750
  Mux : hdlBasic/Mux  inputs=2  en=off  latency=0  precision=Full  arith_type=Unsigned  n_bits=16  bin_pt=14  quantization=Truncate  overflow=Wrap  XmcBlockStatus=1  maskContainerNames=tabcontainer1  block_type=mux  block_config=sysgen:Mux_config
  Mux1 : hdlBasic/Mux  inputs=2  en=off  latency=0  precision=Full  arith_type=Unsigned  n_bits=16  bin_pt=14  quantization=Truncate  overflow=Wrap  XmcBlockStatus=1  maskContainerNames=tabcontainer1  block_type=mux  block_config=sysgen:Mux_config
  Prev1 : hdlBasic/Delay  rst=off  en=off  latency=4  reg_retiming=off  XmcBlockStatus=1  maskContainerNames=group1  block_type=delay  block_config=sysgen:Delay_config
  Register : hdlBasic/Register  init=0  rst=on  en=off  XmcBlockStatus=1  maskContainerNames=tabcontainer1  block_type=register  block_config=sysgen:Register_config
  Register1 : hdlBasic/Register  init=0  rst=on  en=off  XmcBlockStatus=1  maskContainerNames=tabcontainer1  block_type=register  block_config=sysgen:Register_config
  Relational : hdlBasic/Relational  mode=a>b  op_type=Bool  en=on  latency=1  XmcBlockStatus=1  maskContainerNames=tabcontainer1  block_type=relational  block_config=sysgen:Relational_config
  Scope2 : Scope  NumInputPorts=4
  WriteEnable : Outport
  DataMag : Outport  Port=2
  DataINDX : Outport  Port=3
  PeakFound : Outport  Port=4
  Tlast_delayed : Outport  Port=5
  wires:
  FFTValidMask/1 -> Relational/3
  Tlast/1 -> Prev1/1, WriteEnable/1
  Register/1 -> Relational/2, DataMag/1, Mux/2
  Mux/1 -> Register/1
  Register1/1 -> Gateway Out10/1, DataINDX/1, Mux1/2
  FFTIndexTrack/1 -> Gateway Out9/1, Mux1/3
  Mux1/1 -> Register1/1
  Prev1/1 -> Register1/2, Register/2, Tlast_delayed/1
  Gateway Out7/1 -> Scope2/1
  Gateway Out8/1 -> Scope2/2
  Gateway Out9/1 -> Scope2/3
  Gateway Out10/1 -> Scope2/4
  Relational/1 -> Gateway Out8/1, Mux1/1, Mux/1, PeakFound/1
  FFTInput/1 -> Gateway Out7/1, Mux/3, Relational/1

== system RadarSimulinkProjectRev011/RangeProcessing/RX Lowpass Filter ==
  validIN : Inport
  dataIN : Inport  Port=2
  Convert10 : hdlBasic/Convert  gui_display_data_type=Fixed-point  arith_type=Signed (2's comp)  n_bits=32  bin_pt=16  float_type=Single  exp_bits=8  fraction_bits=24  quantization="Round  (unbiased: Even Values)"  overflow=Saturate  en=off  latency=1  pipeline=off  XmcBlockStatus=1  maskContainerNames=group2  block_type=convert  block_config=sysgen:Convert_config  block_width=595  block_height=885
  Convert12 : hdlBasic/Convert  gui_display_data_type=Fixed-point  arith_type=Signed (2's comp)  n_bits=32  bin_pt=16  float_type=Single  exp_bits=8  fraction_bits=24  quantization="Round  (unbiased: Even Values)"  overflow=Saturate  en=off  latency=1  pipeline=off  XmcBlockStatus=1  maskContainerNames=group2  block_type=convert  block_config=sysgen:Convert_config  block_width=595  block_height=885
  Delay : hdlBasic/Delay  rst=off  en=off  latency=413  reg_retiming=off  XmcBlockStatus=1  maskContainerNames=group1  block_type=delay  block_config=sysgen:Delay_config
  Digital FIR Filter6 : hdlBasic/Digital FIR Filter  coeff_source=off  coefficientvector=b1  coeff_calulate=on  coefficient_width=13  coefficient_fractional_bits=13  interpolation_filter_rate=1  decimation_filter_rate=4  fda_coefficientvector=[-0.0024 -0.0042 0.0095 0.0200 -0.0380 -0.0696 0.1374 0.4472 0.4472 0.1374 -0.0696 -0.0380 0.0200 0.0095 -0.0042 -0.0024]  simulation_type=fast_sim  simulation_model=sysgen:fir_macro  XmcBlockStatus=1  maskContainerNames=group1  block_type=fir_macro  block_config=sysgen:fir_macro_config
  Digital FIR Filter7 : hdlBasic/Digital FIR Filter  coeff_source=off  coefficientvector=b2  coeff_calulate=on  coefficient_width=13  coefficient_fractional_bits=13  interpolation_filter_rate=1  decimation_filter_rate=4  fda_coefficientvector=[-0.0024 -0.0042 0.0095 0.0200 -0.0380 -0.0696 0.1374 0.4472 0.4472 0.1374 -0.0696 -0.0380 0.0200 0.0095 -0.0042 -0.0024]  simulation_type=fast_sim  simulation_model=sysgen:fir_macro  XmcBlockStatus=1  maskContainerNames=group1  block_type=fir_macro  block_config=sysgen:fir_macro_config
  Digital FIR Filter8 : hdlBasic/Digital FIR Filter  coeff_source=off  coefficientvector=b3  coeff_calulate=on  coefficient_width=2  coefficient_fractional_bits=2  interpolation_filter_rate=1  decimation_filter_rate=1  fda_coefficientvector=[-0.0024 -0.0042 0.0095 0.0200 -0.0380 -0.0696 0.1374 0.4472 0.4472 0.1374 -0.0696 -0.0380 0.0200 0.0095 -0.0042 -0.0024]  simulation_type=fast_sim  simulation_model=sysgen:fir_macro  XmcBlockStatus=1  maskContainerNames=group1  block_type=fir_macro  block_config=sysgen:fir_macro_config
  tready : Outport
  dataOUT : Outport  Port=2
  wires:
  Digital FIR Filter8/1 -> dataOUT/1
  dataIN/1 -> Digital FIR Filter6/1
  validIN/1 -> Delay/1
  Delay/1 -> tready/1
  Digital FIR Filter6/1 -> Convert10/1
  Convert10/1 -> Digital FIR Filter7/1
  Convert12/1 -> Digital FIR Filter8/1
  Digital FIR Filter7/1 -> Convert12/1

== system RadarSimulinkProjectRev011/RangeProcessing/RX Lowpass Filter1 ==
  dataIN : Inport
  Convert10 : hdlBasic/Convert  gui_display_data_type=Fixed-point  arith_type=Signed (2's comp)  n_bits=32  bin_pt=16  float_type=Single  exp_bits=8  fraction_bits=24  quantization="Round  (unbiased: Even Values)"  overflow=Saturate  en=off  latency=1  pipeline=off  XmcBlockStatus=1  maskContainerNames=group2  block_type=convert  block_config=sysgen:Convert_config  block_width=595  block_height=885
  Convert12 : hdlBasic/Convert  gui_display_data_type=Fixed-point  arith_type=Signed (2's comp)  n_bits=32  bin_pt=16  float_type=Single  exp_bits=8  fraction_bits=24  quantization="Round  (unbiased: Even Values)"  overflow=Saturate  en=off  latency=1  pipeline=off  XmcBlockStatus=1  maskContainerNames=group2  block_type=convert  block_config=sysgen:Convert_config  block_width=595  block_height=885
  Digital FIR Filter6 : hdlBasic/Digital FIR Filter  coeff_source=off  coefficientvector=b1  coeff_calulate=on  coefficient_width=13  coefficient_fractional_bits=13  interpolation_filter_rate=1  decimation_filter_rate=4  fda_coefficientvector=[-0.0024 -0.0042 0.0095 0.0200 -0.0380 -0.0696 0.1374 0.4472 0.4472 0.1374 -0.0696 -0.0380 0.0200 0.0095 -0.0042 -0.0024]  simulation_type=fast_sim  simulation_model=sysgen:fir_macro  XmcBlockStatus=1  maskContainerNames=group1  block_type=fir_macro  block_config=sysgen:fir_macro_config
  Digital FIR Filter7 : hdlBasic/Digital FIR Filter  coeff_source=off  coefficientvector=b2  coeff_calulate=on  coefficient_width=13  coefficient_fractional_bits=13  interpolation_filter_rate=1  decimation_filter_rate=4  fda_coefficientvector=[-0.0024 -0.0042 0.0095 0.0200 -0.0380 -0.0696 0.1374 0.4472 0.4472 0.1374 -0.0696 -0.0380 0.0200 0.0095 -0.0042 -0.0024]  simulation_type=fast_sim  simulation_model=sysgen:fir_macro  XmcBlockStatus=1  maskContainerNames=group1  block_type=fir_macro  block_config=sysgen:fir_macro_config
  Digital FIR Filter8 : hdlBasic/Digital FIR Filter  coeff_source=off  coefficientvector=b3  coeff_calulate=on  coefficient_width=2  coefficient_fractional_bits=2  interpolation_filter_rate=1  decimation_filter_rate=1  fda_coefficientvector=[-0.0024 -0.0042 0.0095 0.0200 -0.0380 -0.0696 0.1374 0.4472 0.4472 0.1374 -0.0696 -0.0380 0.0200 0.0095 -0.0042 -0.0024]  simulation_type=fast_sim  simulation_model=sysgen:fir_macro  XmcBlockStatus=1  maskContainerNames=group1  block_type=fir_macro  block_config=sysgen:fir_macro_config
  dataOUT : Outport
  wires:
  Convert12/1 -> Digital FIR Filter8/1
  Digital FIR Filter6/1 -> Convert10/1
  Digital FIR Filter7/1 -> Convert12/1
  Convert10/1 -> Digital FIR Filter7/1
  Digital FIR Filter8/1 -> dataOUT/1
  dataIN/1 -> Digital FIR Filter6/1

== system RadarSimulinkProjectRev011/RangeProcessing/RX Lowpass Filter2 ==
  dataIN : Inport
  Convert10 : hdlBasic/Convert  gui_display_data_type=Fixed-point  arith_type=Signed (2's comp)  n_bits=32  bin_pt=16  float_type=Single  exp_bits=8  fraction_bits=24  quantization="Round  (unbiased: Even Values)"  overflow=Saturate  en=off  latency=1  pipeline=off  XmcBlockStatus=1  maskContainerNames=group2  block_type=convert  block_config=sysgen:Convert_config  block_width=595  block_height=885
  Convert12 : hdlBasic/Convert  gui_display_data_type=Fixed-point  arith_type=Signed (2's comp)  n_bits=32  bin_pt=16  float_type=Single  exp_bits=8  fraction_bits=24  quantization="Round  (unbiased: Even Values)"  overflow=Saturate  en=off  latency=1  pipeline=off  XmcBlockStatus=1  maskContainerNames=group2  block_type=convert  block_config=sysgen:Convert_config  block_width=595  block_height=885
  Digital FIR Filter6 : hdlBasic/Digital FIR Filter  coeff_source=off  coefficientvector=b1  coeff_calulate=on  coefficient_width=13  coefficient_fractional_bits=13  interpolation_filter_rate=1  decimation_filter_rate=4  fda_coefficientvector=[-0.0024 -0.0042 0.0095 0.0200 -0.0380 -0.0696 0.1374 0.4472 0.4472 0.1374 -0.0696 -0.0380 0.0200 0.0095 -0.0042 -0.0024]  simulation_type=fast_sim  simulation_model=sysgen:fir_macro  XmcBlockStatus=1  maskContainerNames=group1  block_type=fir_macro  block_config=sysgen:fir_macro_config
  Digital FIR Filter7 : hdlBasic/Digital FIR Filter  coeff_source=off  coefficientvector=b2  coeff_calulate=on  coefficient_width=13  coefficient_fractional_bits=13  interpolation_filter_rate=1  decimation_filter_rate=4  fda_coefficientvector=[-0.0024 -0.0042 0.0095 0.0200 -0.0380 -0.0696 0.1374 0.4472 0.4472 0.1374 -0.0696 -0.0380 0.0200 0.0095 -0.0042 -0.0024]  simulation_type=fast_sim  simulation_model=sysgen:fir_macro  XmcBlockStatus=1  maskContainerNames=group1  block_type=fir_macro  block_config=sysgen:fir_macro_config
  Digital FIR Filter8 : hdlBasic/Digital FIR Filter  coeff_source=off  coefficientvector=b3  coeff_calulate=on  coefficient_width=2  coefficient_fractional_bits=2  interpolation_filter_rate=1  decimation_filter_rate=1  fda_coefficientvector=[-0.0024 -0.0042 0.0095 0.0200 -0.0380 -0.0696 0.1374 0.4472 0.4472 0.1374 -0.0696 -0.0380 0.0200 0.0095 -0.0042 -0.0024]  simulation_type=fast_sim  simulation_model=sysgen:fir_macro  XmcBlockStatus=1  maskContainerNames=group1  block_type=fir_macro  block_config=sysgen:fir_macro_config
  dataOUT : Outport
  wires:
  Convert12/1 -> Digital FIR Filter8/1
  Digital FIR Filter6/1 -> Convert10/1
  Digital FIR Filter7/1 -> Convert12/1
  Convert10/1 -> Digital FIR Filter7/1
  Digital FIR Filter8/1 -> dataOUT/1
  dataIN/1 -> Digital FIR Filter6/1

== system RadarSimulinkProjectRev011/RangeProcessing/RX Lowpass Filter3 ==
  dataIN : Inport
  Convert10 : hdlBasic/Convert  gui_display_data_type=Fixed-point  arith_type=Signed (2's comp)  n_bits=32  bin_pt=16  float_type=Single  exp_bits=8  fraction_bits=24  quantization="Round  (unbiased: Even Values)"  overflow=Saturate  en=off  latency=1  pipeline=off  XmcBlockStatus=1  maskContainerNames=group2  block_type=convert  block_config=sysgen:Convert_config  block_width=595  block_height=885
  Convert12 : hdlBasic/Convert  gui_display_data_type=Fixed-point  arith_type=Signed (2's comp)  n_bits=32  bin_pt=16  float_type=Single  exp_bits=8  fraction_bits=24  quantization="Round  (unbiased: Even Values)"  overflow=Saturate  en=off  latency=1  pipeline=off  XmcBlockStatus=1  maskContainerNames=group2  block_type=convert  block_config=sysgen:Convert_config  block_width=595  block_height=885
  Digital FIR Filter6 : hdlBasic/Digital FIR Filter  coeff_source=off  coefficientvector=b1  coeff_calulate=on  coefficient_width=13  coefficient_fractional_bits=13  interpolation_filter_rate=1  decimation_filter_rate=4  fda_coefficientvector=[-0.0024 -0.0042 0.0095 0.0200 -0.0380 -0.0696 0.1374 0.4472 0.4472 0.1374 -0.0696 -0.0380 0.0200 0.0095 -0.0042 -0.0024]  simulation_type=fast_sim  simulation_model=sysgen:fir_macro  XmcBlockStatus=1  maskContainerNames=group1  block_type=fir_macro  block_config=sysgen:fir_macro_config
  Digital FIR Filter7 : hdlBasic/Digital FIR Filter  coeff_source=off  coefficientvector=b2  coeff_calulate=on  coefficient_width=13  coefficient_fractional_bits=13  interpolation_filter_rate=1  decimation_filter_rate=4  fda_coefficientvector=[-0.0024 -0.0042 0.0095 0.0200 -0.0380 -0.0696 0.1374 0.4472 0.4472 0.1374 -0.0696 -0.0380 0.0200 0.0095 -0.0042 -0.0024]  simulation_type=fast_sim  simulation_model=sysgen:fir_macro  XmcBlockStatus=1  maskContainerNames=group1  block_type=fir_macro  block_config=sysgen:fir_macro_config
  Digital FIR Filter8 : hdlBasic/Digital FIR Filter  coeff_source=off  coefficientvector=b3  coeff_calulate=on  coefficient_width=2  coefficient_fractional_bits=2  interpolation_filter_rate=1  decimation_filter_rate=1  fda_coefficientvector=[-0.0024 -0.0042 0.0095 0.0200 -0.0380 -0.0696 0.1374 0.4472 0.4472 0.1374 -0.0696 -0.0380 0.0200 0.0095 -0.0042 -0.0024]  simulation_type=fast_sim  simulation_model=sysgen:fir_macro  XmcBlockStatus=1  maskContainerNames=group1  block_type=fir_macro  block_config=sysgen:fir_macro_config
  dataOUT : Outport
  wires:
  Convert12/1 -> Digital FIR Filter8/1
  Digital FIR Filter6/1 -> Convert10/1
  Digital FIR Filter7/1 -> Convert12/1
  Convert10/1 -> Digital FIR Filter7/1
  Digital FIR Filter8/1 -> dataOUT/1
  dataIN/1 -> Digital FIR Filter6/1
